simulink model "MULT_CYCLE_DDS"  (R2021b)
settings: Solver=VariableStepAuto  StartTime=0.0  StopTime=100000  RelTol=1e-3
values from neighbouring files (symbols this model uses):
  cnt1_max = 255    [mat1.m]
libraries: hdlsllib x4
settings Model: Creator=DELL  LastModifiedBy=DELL

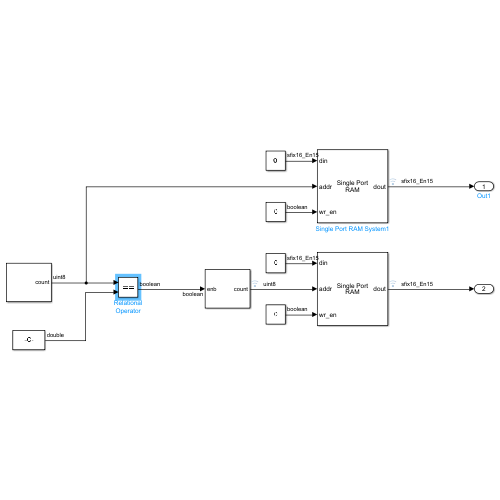
[thumbnail: Simulink's stored preview of the top-level diagram]
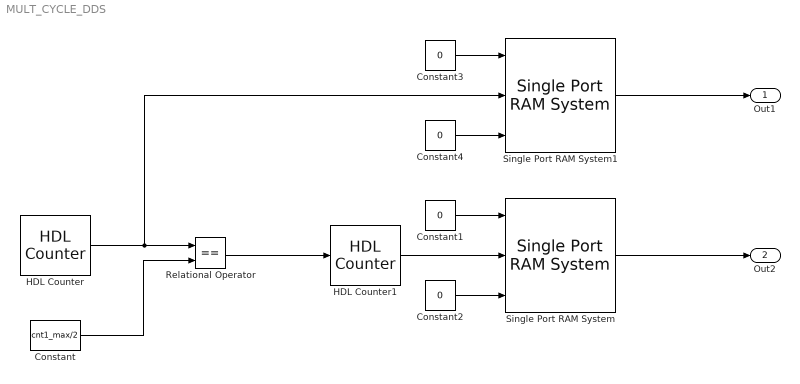
== system MULT_CYCLE_DDS ==
  Constant : Constant  Value=cnt1_max/2  SampleTime=1
  Constant1 : Constant  Value=0  OutDataTypeStr=fixdt(1,16,15)  SampleTime=1
  Constant2 : Constant  Value=0  OutDataTypeStr=boolean  SampleTime=1
  Constant3 : Constant  Value=0  OutDataTypeStr=fixdt(1,16,15)  SampleTime=1
  Constant4 : Constant  Value=0  OutDataTypeStr=boolean  SampleTime=1
  HDL Counter : hdlsllib/Sources/HDL Counter  CountType=Count limited  CountInit=0  CountStep=1  CountMax=cnt1_max  CountFromType=Initial value  CountFrom=0  CountResetPort=off  CountLoadPort=off  CountEnbPort=off  CountDirPort=off  CountHitOutputPort=off  CountDataType=Unsigned  CountWordLen=8  CountFracLen=0  CountSampTime=1
  HDL Counter1 : hdlsllib/Sources/HDL Counter  CountType=Count limited  CountInit=0  CountStep=1  CountMax=cnt2_max  CountFromType=Initial value  CountFrom=0  CountResetPort=off  CountLoadPort=off  CountEnbPort=on  CountDirPort=off  CountHitOutputPort=off  CountDataType=Unsigned  CountWordLen=8  CountFracLen=0  CountSampTime=1
  Relational Operator : RelationalOperator  Operator===  OutDataTypeStr=boolean  RndMeth=Nearest
  Single Port RAM System : hdlsllib/HDL RAMs/Single Port RAM System  RAMType=Single port  WriteOutputValue=New data  RAMInitialValue=sin2_vec  SimulateUsing=Code generation
      settings: SourceProductBaseCode=SL
  Single Port RAM System1 : hdlsllib/HDL RAMs/Single Port RAM System  RAMType=Single port  WriteOutputValue=New data  RAMInitialValue=sin1_vec  SimulateUsing=Code generation
      settings: SourceProductBaseCode=SL
  Out1 : Outport  VectorParamsAs1DForOutWhenUnconnected=off
  Out2 : Outport  Port=2  VectorParamsAs1DForOutWhenUnconnected=off
  wires:
  Constant/1 -> Relational Operator/2
  Relational Operator/1 -> HDL Counter1/1
  HDL Counter1/1 -> Single Port RAM System/2
  Constant1/1 -> Single Port RAM System/1
  Constant2/1 -> Single Port RAM System/3
  HDL Counter/1 -> Single Port RAM System1/2, Relational Operator/1
  Constant4/1 -> Single Port RAM System1/3
  Constant3/1 -> Single Port RAM System1/1
  Single Port RAM System/1 -> Out2/1
  Single Port RAM System1/1 -> Out1/1
